simulink model "PIL_simulation_monitoring_app"  (R2018b)
settings: Solver=FixedStepAuto  StartTime=0.0  StopTime=5  FixedStep=sim_step  RelTol=1e-3
values from neighbouring files (symbols this model uses):
  sim_step = 0.03    [main.m]    (also in vrepUpdateActuator.m)
libraries: pil_lib x1
settings Model: ExtModeTrigDuration=200  Creator=young  LastModifiedBy=computation
settings DataIOCC: SaveOutput=off  SaveTime=off
settings OptimizationCC: DefaultParameterBehavior=Inlined  UseDivisionForNetSlopeComputation=on  UseFloatMulNetSlope=on  InlineInvariantSignals=on  EnhancedBackFolding=on  BooleansAsBitfields=on  PassReuseOutputArgsAs=Individual arguments  StateBitsets=on  DataBitsets=on  ZeroExternalMemoryAtStartup=off  ZeroInternalMemoryAtStartup=off  NoFixptDivByZeroProtection=on  EfficientFloat2IntCast=on  LifeSpan=1  OptimizeBlockOrder=speed  DifferentSizesBufferReuse=on
settings DebuggingCC: ParameterTunabilityLossMsg=error
settings HardwareCC: ProdBitPerPointer=32  ProdBitPerSizeT=32  ProdBitPerPtrDiffT=32  ProdLargestAtomicInteger=Integer  ProdWordSize=32  ProdLongLongMode=on  ProdHWDeviceType=Custom Processor
settings SFSimCC: SimUseLocalCustomCode=off  MATLABDynamicMemAlloc=off
settings RTWCC: SystemTargetFile=CompSOC_ec.tlc  TemplateMakefile=CompSOC_ec.tmf  Description=CompSOC EC Target  GenerateReport=on  RTWUseLocalCustomCode=off  IncludeHyperlinkInReport=on  LaunchReport=on  CreateSILPILBlock=PIL  CodeExecutionProfiling=on  CodeProfilingSaveOptions=AllData  CodeProfilingInstrumentation=detailed  GenerateTraceInfo=on  GenerateTraceReport=on  GenerateTraceReportSl=on  GenerateTraceReportSf=on  GenerateTraceReportEml=on  GenerateWebview=on  GenerateCodeMetricsReport=on
settings CodeAppCC: ForceParamTrailComments=on  IgnoreCustomStorageClasses=off  OperatorAnnotations=on  SimulinkDataObjDesc=on  SFDataObjDesc=on  CustomSymbolStrGlobalVar=rt$N$M  CustomSymbolStrType=$N$M  CustomSymbolStrFcn=$N$M$F  CustomSymbolStrMacro=$N$M  InsertBlockDesc=on
settings STFCustomTargetCC: TargetLibSuffix=.a  TargetLangStandard=C99 (ISO)  MultiwordLength=256  GenerateSampleERTMain=on  IncludeMdlTerminateFcn=off  CombineOutputUpdateFcns=on  CombineSignalStateStructs=on  ERTCustomFileBanners=on  RemoveResetFunc=on  MATLABClassNameForMDSCustomization=Simulink.SoftwareTarget.ERTCustomization  SystemTargetFile=CompSOC_ec.tlc
settings ERTTargetCC: TargetLangStandard=C99 (ISO)  GenerateSampleERTMain=on  ParMdlRefBuildCompliant=off  CompOptLevelCompliant=off  ConcurrentExecutionCompliant=off  IncludeMdlTerminateFcn=off  CombineSignalStateStructs=on  SupportContinuousTime=on  SupportNonInlinedSFcns=on  ModelStepFunctionPrototypeControlCompliant=off  CPPClassGenCompliant=off  UseToolchainInfoCompliant=off  ExtModeStaticAlloc=on  ExtModeStaticAllocSize=9200  ExtModeMexArgs='pato-board.local' 1 9878  InlinedParameterPlacement=NonHierarchical  ERTCustomFileTemplate=CompSOC_ec_file_process.tlc  ERTFilePackagingFormat=CompactWithDataFile

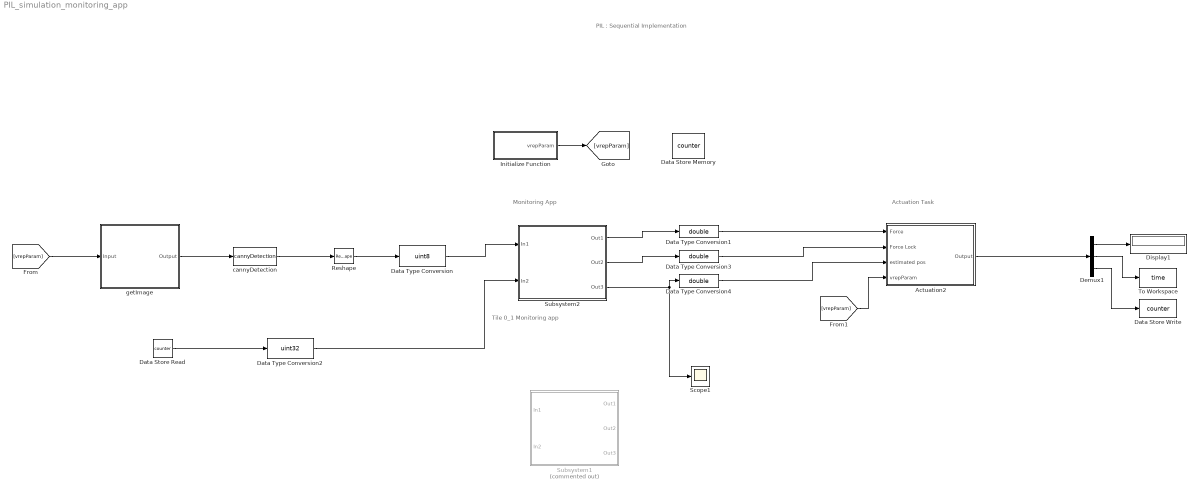
== system PIL_simulation_monitoring_app ==
  note: Tile 0_1 Monitoring app
  note: Actuation Task
  note: Monitoring App
  note: PIL : Sequential Implementation
  Actuation2 : Subsystem
  Data Store Memory : DataStoreMemory  DataStoreName=counter  ReadBeforeWriteMsg=warning  WriteAfterWriteMsg=warning  WriteAfterReadMsg=warning  ShowAdditionalParam=off
  Data Store Read : DataStoreRead  DataStoreName=counter
  Data Store Write : DataStoreWrite  DataStoreName=counter  SampleTime=sim_step
  Data Type Conversion : DataTypeConversion  OutDataTypeStr=uint8
  Data Type Conversion1 : DataTypeConversion  OutDataTypeStr=double
  Data Type Conversion2 : DataTypeConversion  OutDataTypeStr=uint32
  Data Type Conversion3 : DataTypeConversion  OutDataTypeStr=double
  Data Type Conversion4 : DataTypeConversion  OutDataTypeStr=double
  Demux1 : Demux  Outputs=3
  Display1 : Display
  Initialize Function : Subsystem  TreatAsAtomicUnit=on
  Reshape : Reshape
  Scope1 : Scope
  Subsystem1 : Subsystem  Commented=on
  Subsystem2 : Subsystem  DialogController=pil_create_dialog  LoadFcn=|
      | try
      |    if ~strcmp(rtw.pil.getPILVersion, '9.5 (R2018b)_13')
      |       set_param(gcb, 'DialogController', '');
      |       set_param(gcb, 'DialogControllerArgs', '');
      |    end
      | catch e
      |       set_param(gcb, 'DialogController', '');
      |       set_param(gcb, 'DialogControllerArgs', '');
      | end
      mask help: PIL:pil:XILBlockMaskDesc
      mask Display: disp('PIL');
  To Workspace : ToWorkspace  VariableName=time  SampleTime=-1
      settings: Save2DSignal=2-D array (concatenate along first dimension)
  "cannyDetection " : MATLABFcn  MATLABFcn=cannyDetection  Output1D=off
  getImage : Subsystem
  wires:
  [vrepParam] -> getImage/1(Input)
  Initialize Function/1("vrepParam ") -> [vrepParam]
  "cannyDetection "/1 -> Reshape/1
  Reshape/1 -> Data Type Conversion/1
  [vrepParam] -> Actuation2/4(vrepParam)
  Actuation2/1(Output) -> Demux1/1
  Demux1/3 -> Data Store Write/1
  getImage/1(Output) -> "cannyDetection "/1
  Data Store Read/1 -> Data Type Conversion2/1
  Demux1/2 -> To Workspace/1
  Demux1/1 -> Display1/1
  Data Type Conversion3/1 -> Actuation2/2(Force Lock)
  Data Type Conversion4/1 -> Actuation2/3("estimated pos ")
  Data Type Conversion1/1 -> Actuation2/1(Force)
  Subsystem2/3(Out3) -> Scope1/1, Data Type Conversion4/1
  Data Type Conversion/1 -> Subsystem2/1(In1)
  Data Type Conversion2/1 -> Subsystem2/2(In2)
  Subsystem2/1(Out1) -> Data Type Conversion1/1
  Subsystem2/2(Out2) -> Data Type Conversion3/1

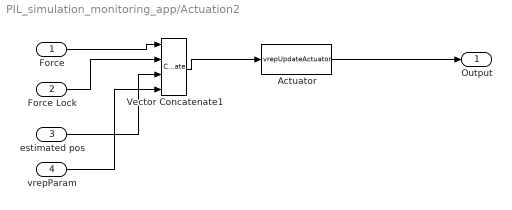
== system PIL_simulation_monitoring_app/Actuation2 ==
  Force : Inport
  Force Lock : Inport  Port=2
  "estimated pos " : Inport  Port=3
  vrepParam : Inport  Port=4
  "Actuator " : MATLABFcn  MATLABFcn=vrepUpdateActuator  OutputDimensions=[1,3]  Output1D=off
  Vector Concatenate1 : Concatenate  NumInputs=4
  Output : Outport
  wires:
  Force/1 -> Vector Concatenate1/1
  Vector Concatenate1/1 -> "Actuator "/1
  "Actuator "/1 -> Output/1
  vrepParam/1 -> Vector Concatenate1/4
  Force Lock/1 -> Vector Concatenate1/2
  "estimated pos "/1 -> Vector Concatenate1/3

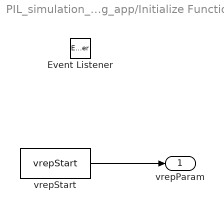
== system PIL_simulation_monitoring_app/Initialize Function ==
  Event Listener : EventListener  DisableCoverage=on  EventName=reset
  "vrepStart " : MATLABFcn  MATLABFcn=vrepStart
  "vrepParam " : Outport
  wires:
  "vrepStart "/1 -> "vrepParam "/1

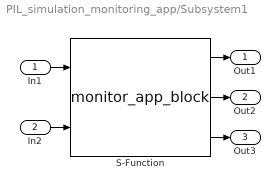
== system PIL_simulation_monitoring_app/Subsystem1 ==
  In1 : Inport
  In2 : Inport  Port=2
  S-Function : S-Function  FunctionName=monitor_app_block  SFunctionDeploymentMode=off  EnableBusSupport=off
  Out1 : Outport
  Out2 : Outport  Port=2
  Out3 : Outport  Port=3
  wires:
  S-Function/1 -> Out1/1
  In1/1 -> S-Function/1
  S-Function/3 -> Out3/1
  S-Function/2 -> Out2/1
  In2/1 -> S-Function/2

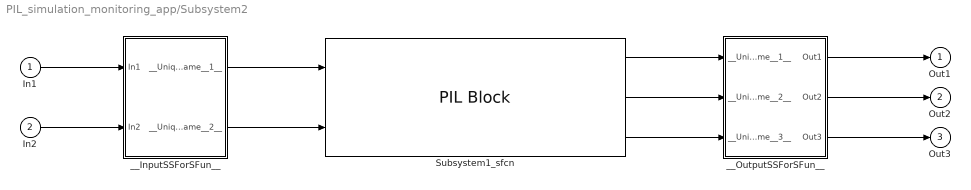
== system PIL_simulation_monitoring_app/Subsystem2 ==
  In1 : Inport
  In2 : Inport  Port=2
  Subsystem1_sfcn : pil_lib/PIL Block  SimulationMode=PIL  IsTopModelPIL=off  CodeDir=/home/computation/5lij0_ECS_Course_2023/PIL_Implementation/PIL_sequential_impl/Subsystem1_CompSOC  AnchorDir=/home/computation/5lij0_ECS_Course_2023/PIL_Implementation/PIL_sequential_impl  ConfigName=CompSOC connectivity config using serial  XrelIsTopModelCode=on  XrelIsReusable=off  XrelDWorkNames={}  XrelDWorkTypes={}  XrelModelArgVals={}  XrelOrderedParamNames={}
  __InputSSForSFun__ : Subsystem
  __OutputSSForSFun__ : Subsystem
  Out1 : Outport
  Out2 : Outport  Port=2
  Out3 : Outport  Port=3
  wires:
  __OutputSSForSFun__/3(Out3) -> Out3/1
  __OutputSSForSFun__/2(Out2) -> Out2/1
  __OutputSSForSFun__/1(Out1) -> Out1/1
  Subsystem1_sfcn/3 -> __OutputSSForSFun__/3(__UniqueInportName__3__)
  Subsystem1_sfcn/2 -> __OutputSSForSFun__/2(__UniqueInportName__2__)
  Subsystem1_sfcn/1 -> __OutputSSForSFun__/1(__UniqueInportName__1__)
  __InputSSForSFun__/2(__UniqueOutportName__2__) -> Subsystem1_sfcn/2
  __InputSSForSFun__/1(__UniqueOutportName__1__) -> Subsystem1_sfcn/1
  In2/1 -> __InputSSForSFun__/2(In2)
  In1/1 -> __InputSSForSFun__/1(In1)

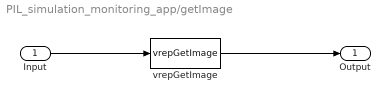
== system PIL_simulation_monitoring_app/getImage ==
  Input : Inport
  vrepGetImage : MATLABFcn  MATLABFcn=vrepGetImage  OutputDimensions=[142,88]  Output1D=off
  Output : Outport
  wires:
  vrepGetImage/1 -> Output/1
  Input/1 -> vrepGetImage/1

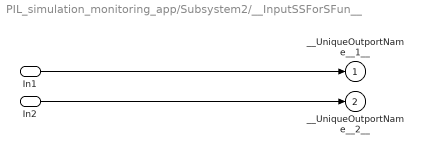
== system PIL_simulation_monitoring_app/Subsystem2/__InputSSForSFun__ ==
  In1 : Inport
  In2 : Inport  Port=2
  __UniqueOutportName__1__ : Outport
  __UniqueOutportName__2__ : Outport  Port=2
  wires:
  In2/1 -> __UniqueOutportName__2__/1
  In1/1 -> __UniqueOutportName__1__/1

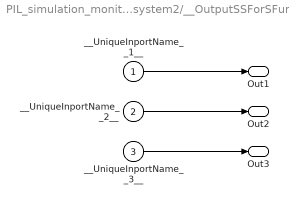
== system PIL_simulation_monitoring_app/Subsystem2/__OutputSSForSFun__ ==
  __UniqueInportName__1__ : Inport
  __UniqueInportName__2__ : Inport  Port=2
  __UniqueInportName__3__ : Inport  Port=3
  Out1 : Outport
  Out2 : Outport  Port=2
  Out3 : Outport  Port=3
  wires:
  __UniqueInportName__3__/1 -> Out3/1
  __UniqueInportName__2__/1 -> Out2/1
  __UniqueInportName__1__/1 -> Out1/1
